simulink model "Ramp_Function"  (R2025b)
settings: Solver=ode4  StartTime=0.0  StopTime=10.0  RelTol=1e-3
settings Model: Creator=Torstein  LastModifiedBy=Torstein

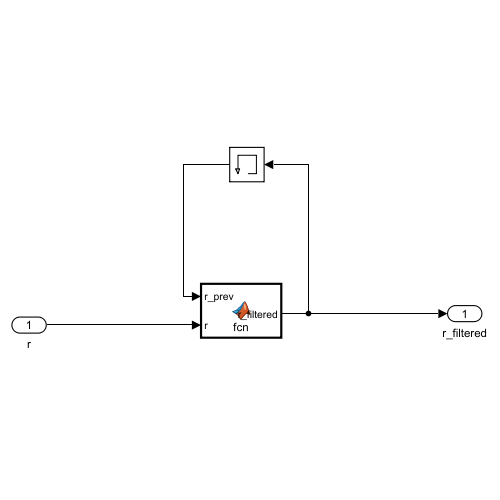
[thumbnail: Simulink's stored preview of the top-level diagram]
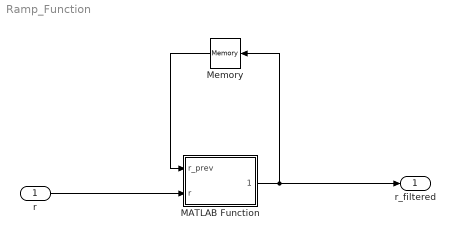
== system Ramp_Function ==
  r : Inport
  MATLAB Function : MATLAB Function  TreatAsAtomicUnit=on
  Memory : Memory
  r_filtered : Outport
  wires:
  Memory/1 -> MATLAB Function/1(r_prev)
  MATLAB Function/1(r_filtered) -> Memory/1, r_filtered/1
  r/1 -> MATLAB Function/2(r)

== matlab function Ramp_Function/MATLAB Function ==
  data: r_prev input; r input; r_filtered output
function r_filtered = fcn(r_prev, r)

if r_prev == 0
    r_prev = r;
end
max_diff = 0.01;
diff = r - r_prev;
if abs(diff) > max_diff
    r_filtered = r_prev + sign(diff) * max_diff;
else
    r_filtered = r;
end
